simulink model "simulink_aircraft_simulation"  (R2016b)
settings: Solver=VariableStepAuto  StartTime=0.0  StopTime=TF  RelTol=1e-3
values from neighbouring files (symbols this model uses):
  a = 6378137.0    (= 6378137)    [InitialConditions.m]
  e = 0.081819190842622    (= 0.0818191908426)    [InitialConditions.m]
  latitude0 = deg2rad(40.416775)    [InitialConditions.m]
  longitude0 = deg2rad(-3.70390)    [InitialConditions.m]
  pNED = [0 ... (first row only)    [InitialConditions.m]
  TF = 60    [InitialConditions.m]
  u1max = 25*pi/180    (= 0.436332312999)    [InitialConditions.m]
  u1min = -25*pi/180    (= -0.436332312999)    [InitialConditions.m]
  u2max = 10*pi/180    (= 0.174532925199)    [InitialConditions.m]
  u2min = -25*pi/180    (= -0.436332312999)    [InitialConditions.m]
  u3max = 30*pi/180    (= 0.523598775598)    [InitialConditions.m]
  u3min = -30*pi/180    (= -0.523598775598)    [InitialConditions.m]
  u4max = 10*pi/180    (= 0.174532925199)    [InitialConditions.m]
  u4min = 0.5*pi/180    (= 0.00872664625997)    [InitialConditions.m]
  u5max = 10*pi/180    (= 0.174532925199)    [InitialConditions.m]
  u5min = 0.5*pi/180    (= 0.00872664625997)    [InitialConditions.m]
  x0 = [85 ... (first row only)    [InitialConditions.m]
undefined symbols (not defined in the file or in its folder): Aircraft_model
libraries: simulink x5, aerolibutil x2, aerolibfltsims x2, vrlib x1
settings Model: Creator=alexzongo  LastModifiedBy=alexzongo

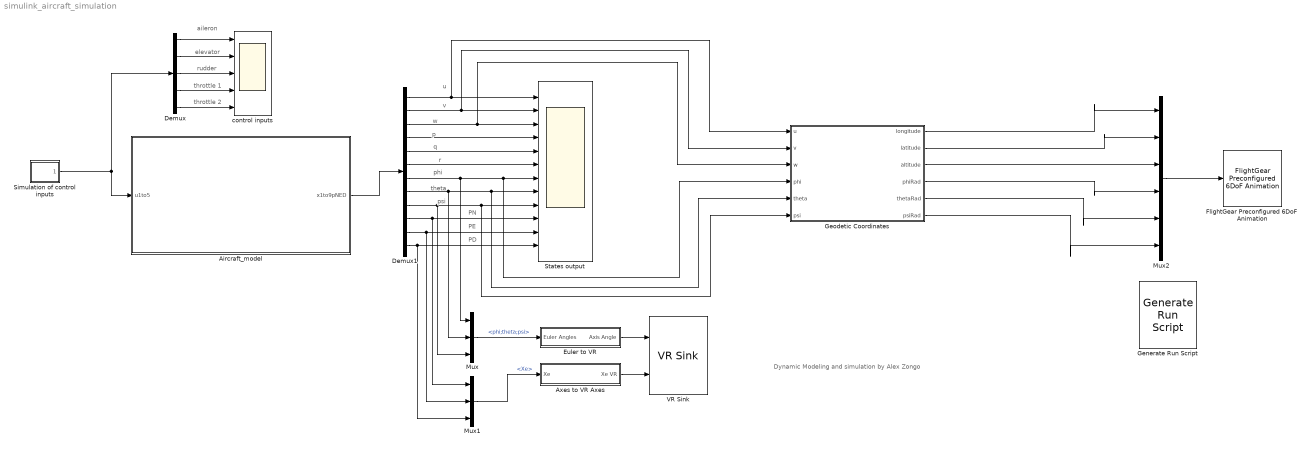
== system simulink_aircraft_simulation ==
  note: Dynamic Modeling and simulation
      | by Alex Zongo
  note: PD
  note: PE
  note: PN
  note: psi
  note: theta
  note: phi
  note: r
  note: q
  note: p
  note: w
  note: v
  note: u
  note: throttle 2
  note: throttle 1
  note: rudder
  note: elevator
  note: aileron
  Aircraft_model : Subsystem
      mask Display: image('Screen Shot 2020-12-07 at 8.20.08 PM.png');
  Axes to VR Axes : Subsystem
  Demux : Demux  Outputs=5
  Demux1 : Demux  Outputs=12
  Euler to VR : Subsystem
  FlightGear Preconfigured 6DoF Animation : aerolibfltsims/FlightGear Preconfigured 6DoF Animation  xFlightGearVersion=v2016.1  DestinationIpAddress=127.0.0.1  DestinationPort=5502  SampleTime=1/30
  Generate Run Script : aerolibfltsims/Generate Run Script  OutputFileName=runfg.sh  FlightGearBaseDirectory=/Users/alexzongo/Applications  GeometryModelName=A380  DestinationPort=5502  OriginAddress=127.0.0.1  OriginPort=5505  LocalAddress=127.0.0.1  AirportId=KSFO  RunwayId=10L  InitialAltitude=7224  InitialHeading=113  OffsetDistance=4.72  OffsetAzimuth=0  GenerateFile=off  Architecture=Mac  dataFlow=Send
  Geodetic Coordinates : Subsystem
  Mux : Mux  Inputs=3
  Mux1 : Mux  Inputs=3
  Mux2 : Mux  Inputs=6
  Simulation of control inputs : Subsystem
  States output : Scope  NumInputPorts=12
  VR Sink : vrlib/VR Sink  InstantiateOnLoad=on  SampleTime=0.1  ViewEnable=on  RemoteChange=off  RemoteView=off  FieldsWritten=HL20.rotation.4.1.1.double#HL20.translation.3.1.1.double  WorldFileName=aeroblk_HL20.wrl  WorldDescription=aeroblk_HL20  AutoView=on  VideoDimensions=[]  AllowVariableSize=off
  control inputs : Scope  NumInputPorts=5
  wires:
  Aircraft_model/1(x1to9pNED) -> Demux1/1
  Simulation of control inputs/1(simUin) -> Demux/1, Aircraft_model/1(u1to5)
  Demux/1 -> control inputs/1
  Demux/2 -> control inputs/2
  Demux/3 -> control inputs/3
  Demux/4 -> control inputs/4
  Demux/5 -> control inputs/5
  Demux1/1 -> Geodetic Coordinates/1(u), States output/1
  Demux1/2 -> Geodetic Coordinates/2(v), States output/2
  Demux1/3 -> Geodetic Coordinates/3(w), States output/3
  Demux1/4 -> States output/4
  Demux1/5 -> States output/5
  Demux1/6 -> States output/6
  Demux1/7 -> Mux/1, Geodetic Coordinates/4(phi), States output/7
  Demux1/8 -> Geodetic Coordinates/5(theta), States output/8, Mux/2
  Demux1/9 -> Mux/3, Geodetic Coordinates/6(psi), States output/9
  Demux1/10 -> Mux1/1, States output/10
  Demux1/12 -> Mux1/3, States output/12
  Mux/1 -> Euler to VR/1(Euler Angles)  "<phi;theta;psi>"
  Mux1/1 -> Axes to VR Axes/1(Xe)  "<Xe>"
  Euler to VR/1(Axis Angle) -> VR Sink/1
  Axes to VR Axes/1(Xe VR) -> VR Sink/2
  Demux1/11 -> Mux1/2, States output/11
  Mux2/1 -> FlightGear Preconfigured 6DoF Animation/1
  Geodetic Coordinates/1(longitude) -> Mux2/1
  Geodetic Coordinates/2(latitude) -> Mux2/2
  Geodetic Coordinates/3(altitude) -> Mux2/3
  Geodetic Coordinates/4(phiRad) -> Mux2/4
  Geodetic Coordinates/5(thetaRad) -> Mux2/5
  Geodetic Coordinates/6(psiRad) -> Mux2/6

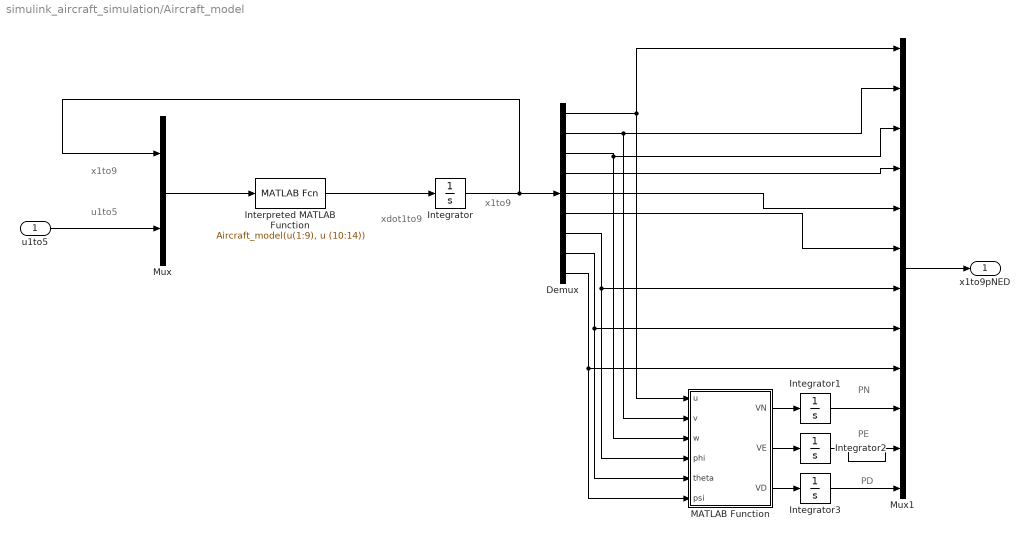
== system simulink_aircraft_simulation/Aircraft_model ==
  note: PD
  note: PE
  note: PN
  note: x1to9
  note: u1to5
  note: x1to9
  note: xdot1to9
  u1to5 : Inport
  Demux : Demux  Outputs=9
  Integrator : Integrator  InitialCondition=x0
  Integrator1 : Integrator  InitialCondition=pNED(1)
  Integrator2 : Integrator  InitialCondition=pNED(2)
  Integrator3 : Integrator  InitialCondition=pNED(3)
  Interpreted MATLAB Function : MATLABFcn  MATLABFcn=Aircraft_model(u(1:9), u (10:14))
  MATLAB Function : MATLAB Function  TreatAsAtomicUnit=on
  Mux : Mux  Inputs=2
  Mux1 : Mux  Inputs=12
  x1to9pNED : Outport
  wires:
  Interpreted MATLAB Function/1 -> Integrator/1
  Integrator/1 -> Demux/1, Mux/1
  Mux/1 -> Interpreted MATLAB Function/1
  u1to5/1 -> Mux/2
  Demux/1 -> Mux1/1, MATLAB Function/1(u)
  Demux/2 -> Mux1/2, MATLAB Function/2(v)
  Demux/3 -> Mux1/3, MATLAB Function/3(w)
  Demux/7 -> Mux1/7, MATLAB Function/4(phi)
  Demux/8 -> Mux1/8, MATLAB Function/5(theta)
  Demux/9 -> Mux1/9, MATLAB Function/6(psi)
  MATLAB Function/3(VD) -> Integrator3/1
  MATLAB Function/2(VE) -> Integrator2/1
  MATLAB Function/1(VN) -> Integrator1/1
  Integrator1/1 -> Mux1/10
  Integrator2/1 -> Mux1/11
  Integrator3/1 -> Mux1/12
  Demux/6 -> Mux1/6
  Demux/5 -> Mux1/5
  Demux/4 -> Mux1/4
  Mux1/1 -> x1to9pNED/1

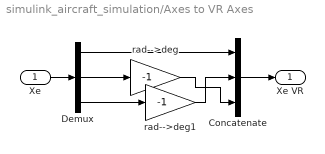
== system simulink_aircraft_simulation/Axes to VR Axes ==
  Xe : Inport
  Concatenate : Concatenate  NumInputs=3
  Demux : Demux  Outputs=3
  rad-->deg : Gain  Gain=-1  SaturateOnIntegerOverflow=on  OutDataTypeStr=Inherit: Same as input  ParamDataTypeStr=Inherit: Same as input
  rad-->deg1 : Gain  Gain=-1  SaturateOnIntegerOverflow=on  OutDataTypeStr=Inherit: Same as input  ParamDataTypeStr=Inherit: Same as input
  Xe VR : Outport
  wires:
  Xe/1 -> Demux/1
  Demux/1 -> Concatenate/1
  Demux/2 -> rad-->deg/1
  Demux/3 -> rad-->deg1/1
  Concatenate/1 -> Xe VR/1
  rad-->deg1/1 -> Concatenate/2
  rad-->deg/1 -> Concatenate/3

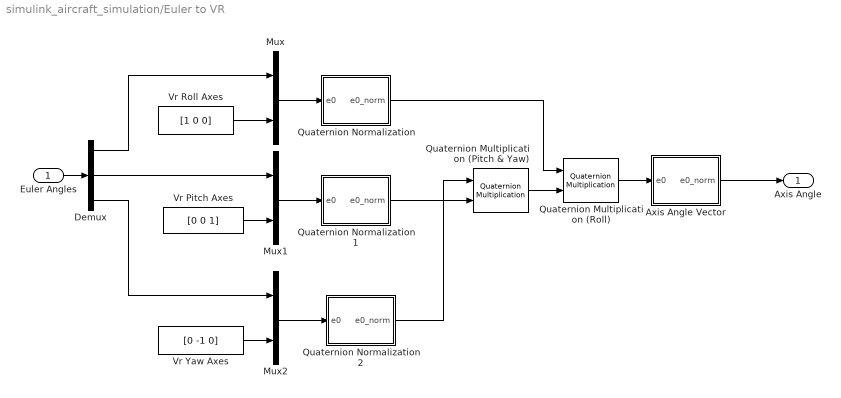
== system simulink_aircraft_simulation/Euler to VR ==
  Euler Angles : Inport
  Axis Angle Vector : Subsystem
  Demux : Demux  Outputs=3
  Mux : Mux  Inputs=2
  Mux1 : Mux  Inputs=2
  Mux2 : Mux  Inputs=2
  Quaternion Multiplication (Pitch & Yaw) : aerolibutil/Quaternion Multiplication
  Quaternion Multiplication (Roll) : aerolibutil/Quaternion Multiplication
  Quaternion Normalization : Subsystem
  Quaternion Normalization1 : Subsystem
  Quaternion Normalization2 : Subsystem
  Vr Pitch Axes : Constant  Value=[0 0 1]
  Vr Roll Axes : Constant  Value=[1 0 0]
  Vr Yaw Axes : Constant  Value=[0 -1 0]
  Axis Angle : Outport
  wires:
  Quaternion Multiplication (Roll)/1 -> Axis Angle Vector/1(e0)
  Quaternion Multiplication (Pitch & Yaw)/1 -> Quaternion Multiplication (Roll)/2
  Axis Angle Vector/1(e0_norm) -> Axis Angle/1
  Quaternion Normalization/1(e0_norm) -> Quaternion Multiplication (Roll)/1
  Quaternion Normalization2/1(e0_norm) -> Quaternion Multiplication (Pitch & Yaw)/1
  Quaternion Normalization1/1(e0_norm) -> Quaternion Multiplication (Pitch & Yaw)/2
  Mux2/1 -> Quaternion Normalization2/1(e0)
  Mux1/1 -> Quaternion Normalization1/1(e0)
  Mux/1 -> Quaternion Normalization/1(e0)
  Demux/3 -> Mux2/1
  Vr Yaw Axes/1 -> Mux2/2
  Demux/2 -> Mux1/1
  Vr Pitch Axes/1 -> Mux1/2
  Demux/1 -> Mux/1
  Vr Roll Axes/1 -> Mux/2
  Euler Angles/1 -> Demux/1

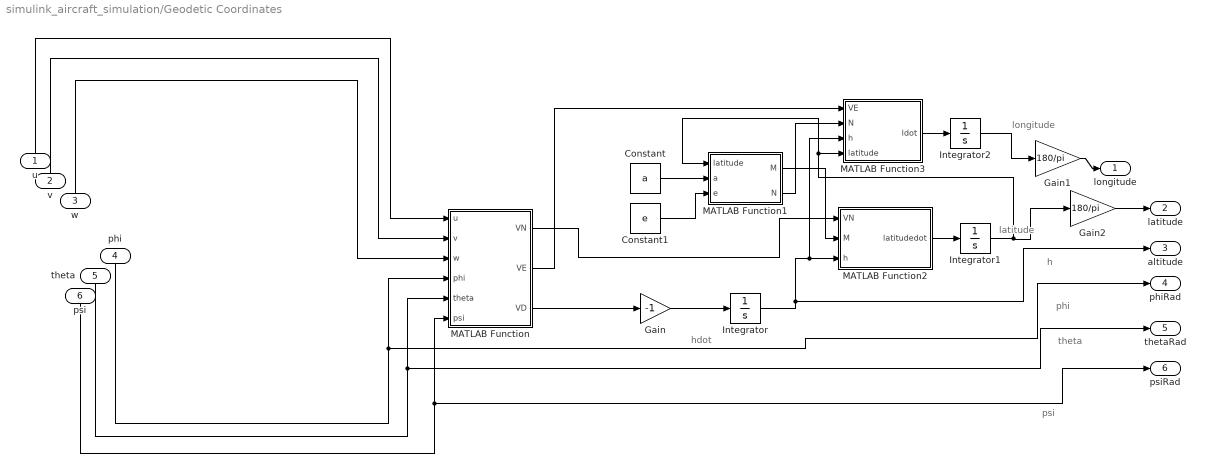
== system simulink_aircraft_simulation/Geodetic Coordinates ==
  note: psi
  note: theta
  note: phi
  note: longitude
  note: latitude
  note: h
  note: hdot
  u : Inport
  v : Inport  Port=2
  w : Inport  Port=3
  phi : Inport  Port=4
  theta : Inport  Port=5
  psi : Inport  Port=6
  Constant : Constant  Value=a
  Constant1 : Constant  Value=e
  Gain : Gain  Gain=-1
  Gain1 : Gain  Gain=180/pi
  Gain2 : Gain  Gain=180/pi
  Integrator : Integrator  InitialCondition=-pNED(3)
  Integrator1 : Integrator  InitialCondition=latitude0
  Integrator2 : Integrator  InitialCondition=longitude0
  MATLAB Function : MATLAB Function  TreatAsAtomicUnit=on
  MATLAB Function1 : MATLAB Function  TreatAsAtomicUnit=on
  MATLAB Function2 : MATLAB Function  TreatAsAtomicUnit=on
  MATLAB Function3 : MATLAB Function  TreatAsAtomicUnit=on
  longitude : Outport
  latitude : Outport  Port=2
  altitude : Outport  Port=3
  phiRad : Outport  Port=4
  thetaRad : Outport  Port=5
  psiRad : Outport  Port=6
  wires:
  Gain/1 -> Integrator/1
  MATLAB Function/3(VD) -> Gain/1
  MATLAB Function/1(VN) -> MATLAB Function2/1(VN)
  MATLAB Function/2(VE) -> MATLAB Function3/1(VE)
  psi/1 -> psiRad/1, MATLAB Function/6(psi)
  Constant1/1 -> MATLAB Function1/3(e)
  Constant/1 -> MATLAB Function1/2(a)
  phi/1 -> phiRad/1, MATLAB Function/4(phi)
  theta/1 -> thetaRad/1, MATLAB Function/5(theta)
  MATLAB Function3/1(ldot) -> Integrator2/1
  u/1 -> MATLAB Function/1(u)
  v/1 -> MATLAB Function/2(v)
  Integrator/1 -> altitude/1, MATLAB Function3/3(h), MATLAB Function2/3(h)
  MATLAB Function2/1(latitudedot) -> Integrator1/1
  Integrator1/1 -> Gain2/1, MATLAB Function3/4(latitude), MATLAB Function1/1(latitude)
  w/1 -> MATLAB Function/3(w)
  MATLAB Function1/2(N) -> MATLAB Function3/2(N)
  MATLAB Function1/1(M) -> MATLAB Function2/2(M)
  Gain1/1 -> longitude/1
  Integrator2/1 -> Gain1/1
  Gain2/1 -> latitude/1

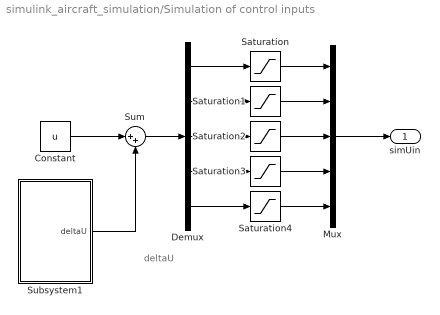
== system simulink_aircraft_simulation/Simulation of control inputs ==
  note: deltaU
  Constant : Constant  Value=u
  Demux : Demux  Outputs=5
  Mux : Mux  Inputs=5
  Saturation : Saturate  UpperLimit=u1max  LowerLimit=u1min
  Saturation1 : Saturate  UpperLimit=u2max  LowerLimit=u2min
  Saturation2 : Saturate  UpperLimit=u3max  LowerLimit=u3min
  Saturation3 : Saturate  UpperLimit=u4max  LowerLimit=u4min
  Saturation4 : Saturate  UpperLimit=u5max  LowerLimit=u5min
  Subsystem1 : Subsystem
  Sum : Sum  Inputs=|++
  simUin : Outport
  wires:
  Subsystem1/1(deltaU) -> Sum/2
  Constant/1 -> Sum/1
  Sum/1 -> Demux/1
  Demux/1 -> Saturation/1
  Demux/2 -> Saturation1/1
  Demux/3 -> Saturation2/1
  Demux/4 -> Saturation3/1
  Demux/5 -> Saturation4/1
  Saturation/1 -> Mux/1
  Saturation1/1 -> Mux/2
  Saturation2/1 -> Mux/3
  Saturation3/1 -> Mux/4
  Saturation4/1 -> Mux/5
  Mux/1 -> simUin/1

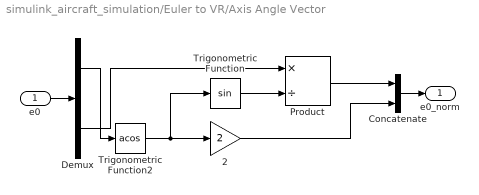
== system simulink_aircraft_simulation/Euler to VR/Axis Angle Vector ==
  e0 : Inport
  2 : Gain  Gain=2  SaturateOnIntegerOverflow=on  OutDataTypeStr=Inherit: Same as input  ParamDataTypeStr=Inherit: Same as input
  Concatenate : Concatenate
  Demux : Demux  Outputs=[1 3 ]
  Product : Product  Inputs=*/  SaturateOnIntegerOverflow=on  InputSameDT=on  OutDataTypeStr=Inherit: Same as first input
  Trigonometric Function : Trigonometry
  Trigonometric Function2 : Trigonometry  Operator=acos
  e0_norm : Outport
  wires:
  Demux/1 -> Trigonometric Function2/1
  Demux/2 -> Product/1
  Concatenate/1 -> e0_norm/1
  Product/1 -> Concatenate/1
  2/1 -> Concatenate/2
  Trigonometric Function/1 -> Product/2
  Trigonometric Function2/1 -> Trigonometric Function/1, 2/1
  e0/1 -> Demux/1

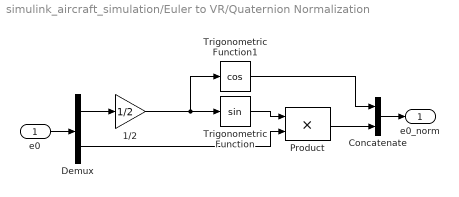
== system simulink_aircraft_simulation/Euler to VR/Quaternion Normalization ==
  e0 : Inport
  1/2 : Gain  Gain=1/2  SaturateOnIntegerOverflow=on  OutDataTypeStr=Inherit: Same as input  ParamDataTypeStr=Inherit: Same as input
  Concatenate : Concatenate
  Demux : Demux  Outputs=[1 3]
  Product : Product  SaturateOnIntegerOverflow=on  InputSameDT=on  OutDataTypeStr=Inherit: Same as first input
  Trigonometric Function : Trigonometry
  Trigonometric Function1 : Trigonometry  Operator=cos
  e0_norm : Outport
  wires:
  Trigonometric Function1/1 -> Concatenate/1
  Demux/2 -> Product/2
  Demux/1 -> 1/2/1
  Concatenate/1 -> e0_norm/1
  Product/1 -> Concatenate/2
  Trigonometric Function/1 -> Product/1
  1/2/1 -> Trigonometric Function1/1, Trigonometric Function/1
  e0/1 -> Demux/1

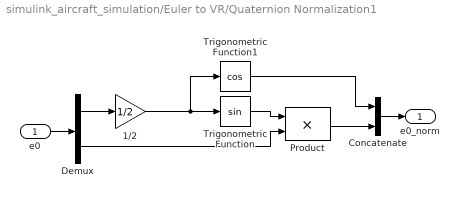
== system simulink_aircraft_simulation/Euler to VR/Quaternion Normalization1 ==
  e0 : Inport
  1/2 : Gain  Gain=1/2  SaturateOnIntegerOverflow=on  OutDataTypeStr=Inherit: Same as input  ParamDataTypeStr=Inherit: Same as input
  Concatenate : Concatenate
  Demux : Demux  Outputs=[1 3]
  Product : Product  SaturateOnIntegerOverflow=on  InputSameDT=on  OutDataTypeStr=Inherit: Same as first input
  Trigonometric Function : Trigonometry
  Trigonometric Function1 : Trigonometry  Operator=cos
  e0_norm : Outport
  wires:
  e0/1 -> Demux/1
  1/2/1 -> Trigonometric Function/1, Trigonometric Function1/1
  Trigonometric Function/1 -> Product/1
  Product/1 -> Concatenate/2
  Concatenate/1 -> e0_norm/1
  Demux/1 -> 1/2/1
  Demux/2 -> Product/2
  Trigonometric Function1/1 -> Concatenate/1

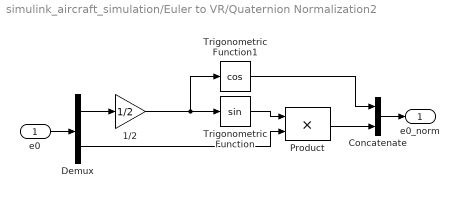
== system simulink_aircraft_simulation/Euler to VR/Quaternion Normalization2 ==
  e0 : Inport
  1/2 : Gain  Gain=1/2  SaturateOnIntegerOverflow=on  OutDataTypeStr=Inherit: Same as input  ParamDataTypeStr=Inherit: Same as input
  Concatenate : Concatenate
  Demux : Demux  Outputs=[1 3]
  Product : Product  SaturateOnIntegerOverflow=on  InputSameDT=on  OutDataTypeStr=Inherit: Same as first input
  Trigonometric Function : Trigonometry
  Trigonometric Function1 : Trigonometry  Operator=cos
  e0_norm : Outport
  wires:
  Trigonometric Function1/1 -> Concatenate/1
  Demux/2 -> Product/2
  Demux/1 -> 1/2/1
  Concatenate/1 -> e0_norm/1
  Product/1 -> Concatenate/2
  Trigonometric Function/1 -> Product/1
  1/2/1 -> Trigonometric Function1/1, Trigonometric Function/1
  e0/1 -> Demux/1

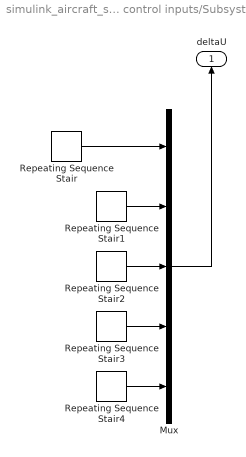
== system simulink_aircraft_simulation/Simulation of control inputs/Subsystem1 ==
  Mux : Mux  Inputs=5
  Repeating Sequence Stair : simulink/Sources/Repeating Sequence Stair  OutValues="[10*pi/180 0 0 0  -10*pi/180 0 0 0 5*pi/180 0 0 0 -5*pi/180 ].'"  tsamp=TF/10  OutMin=[]  OutMax=[]  OutDataTypeStr=double  OutputDataTypeScalingMode=double  OutDataType=fixdt(0,8)  ConRadixGroup=Best Precision: Vector-wise  OutScaling=2^-12
  Repeating Sequence Stair1 : simulink/Sources/Repeating Sequence Stair  OutValues=[0 0 0 0 0 0 0 5*pi/180 0 0 0 -5*pi/180 0 0 0].'  tsamp=TF/10  OutMin=[]  OutMax=[]  OutDataTypeStr=double  OutputDataTypeScalingMode=double  OutDataType=fixdt(0,8)  ConRadixGroup=Best Precision: Vector-wise  OutScaling=2^-12
  Repeating Sequence Stair2 : simulink/Sources/Repeating Sequence Stair  OutValues=[ 0 0 0 0 0 0 0 0 0 0 0 0 0 0 0 0 0 0 0 5*pi/180 0 0 0 -5*pi/180 0 0 0].'  tsamp=TF/10  OutMin=[]  OutMax=[]  OutDataTypeStr=double  OutputDataTypeScalingMode=double  OutDataType=fixdt(0,8)  ConRadixGroup=Best Precision: Vector-wise  OutScaling=2^-12
  Repeating Sequence Stair3 : simulink/Sources/Repeating Sequence Stair  OutValues=[0 0 0 0 0 0 0 5*pi/180 0 0 0 -5*pi/180 0 0 0].'  tsamp=TF/10  OutMin=[]  OutMax=[]  OutDataTypeStr=double  OutputDataTypeScalingMode=double  OutDataType=fixdt(0,8)  ConRadixGroup=Best Precision: Vector-wise  OutScaling=2^-12
  Repeating Sequence Stair4 : simulink/Sources/Repeating Sequence Stair  OutValues=[0 0 0 0 0 0 0 5*pi/180 0 0 0 -5*pi/180 0 0 0].'  tsamp=TF/10  OutMin=[]  OutMax=[]  OutDataTypeStr=double  OutputDataTypeScalingMode=double  OutDataType=fixdt(0,8)  ConRadixGroup=Best Precision: Vector-wise  OutScaling=2^-12
  deltaU : Outport
  wires:
  Repeating Sequence Stair1/1 -> Mux/2
  Mux/1 -> deltaU/1
  Repeating Sequence Stair4/1 -> Mux/5
  Repeating Sequence Stair3/1 -> Mux/4
  Repeating Sequence Stair2/1 -> Mux/3
  Repeating Sequence Stair/1 -> Mux/1

== matlab function simulink_aircraft_simulation/Geodetic Coordinates/MATLAB Function ==
  data: u input; VN output; v input; w input; phi input; theta input; psi input; VE output; VD output
function [VN, VE, VD] = fcn(u, v, w, phi, theta, psi)

c1v=[cos(psi) sin(psi) 0; -sin(psi) cos(psi) 0; 0 0 1];
c21=[cos(theta) 0 -sin(theta); 0 1 0; sin(theta) 0 cos(theta)];
cb2=[1 0 0; 0 cos(phi) sin(phi); 0 -sin(phi) cos(phi)];

cbv=cb2*c21*c1v;
V_b=[u; v; w];
V_v = cbv'*V_b;
VN=V_v(1);
VE = V_v(2);
VD = V_v(3);

== matlab function simulink_aircraft_simulation/Aircraft_model/MATLAB Function ==
  data: u input; VN output; v input; w input; phi input; theta input; psi input; VE output; VD output
function [VN, VE, VD] = fcn(u, v, w, phi, theta, psi)

c1v=[cos(psi) sin(psi) 0; -sin(psi) cos(psi) 0; 0 0 1];
c21=[cos(theta) 0 -sin(theta); 0 1 0; sin(theta) 0 cos(theta)];
cb2=[1 0 0; 0 cos(phi) sin(phi); 0 -sin(phi) cos(phi)];

cbv=cb2*c21*c1v;
V_b=[u; v; w];
V_v = cbv'*V_b;
VN=V_v(1);
VE = V_v(2);
VD = V_v(3);

== matlab function simulink_aircraft_simulation/Geodetic Coordinates/MATLAB Function1 ==
  data: latitude input; M output; a input; e input; N output
function [M, N] = fcn(latitude, a, e)

M = (a*(1-e^2))/((1-(e*sin(latitude))^2)^1.5);
N = a/((1-(e*sin(latitude))^2)^0.5);

== matlab function simulink_aircraft_simulation/Geodetic Coordinates/MATLAB Function2 ==
  data: VN input; latitudedot output; M input; h input
function latitudedot  = fcn(VN, M, h)

latitudedot = VN/(M+h);

== matlab function simulink_aircraft_simulation/Geodetic Coordinates/MATLAB Function3 ==
  data: VE input; ldot output; N input; h input; latitude input
function ldot = fcn(VE, N, h, latitude)

ldot = VE/((N+h)*cos(latitude));
